simulink model "Parametrica"  (R2020b)
settings: Solver=VariableStepAuto  StartTime=0.0  StopTime=Smi.general.simulation_time  FixedStep=0.001  MaxStep=0.001  RelTol=1e-3  AbsTol=1e-3  EnableMultiTasking=on
undefined symbols (not defined in the file or in its folder): Smi, X, Y, Z
libraries: sm_lib x755, nesl_utility x196, simulink x8, dspsrcs4 x8, cstblocks x8
(part 6 of 26)

== system Parametrica/FIXED CHASSIS/WORLD ==
  Mechanism Configuration : sm_lib/Utilities/Mechanism Configuration  UniformGravity=Constant  GravityVector=[0 0 -9.80665]  GravityVectorUnits=m/s^2  GravityUnits=m/s^2  LinearizationDelta=0.001  JointModeTransitionNonlinearIterations=2
      settings: SourceProductName=Multibody
  Solver Configuration : nesl_utility/Solver Configuration  PhysicalDomain=network_engine_domain  SubClassName=solver  LeftPortType=input  RightPortType=generic  Tones=[]  Harmonics=[]  SimulateNoise=off  Profile=off  UseLocalSampling=off  EnableSwitchedLinearOptims=on  FrequencyDomain=off  UseCCode=off  RelTol=0.001  AbsTol=1e-06  MinStep=1e-09  ToWorkspace=off  RevertToSquareIcSolve=off  NumHomotopyIterations=100  PhasorMode=off  PhasorModeNumHarmonics=1  DoDC=off  ResidualTolerance=1e-09  UseLocalSolver=off  LocalSolverChoice=NE_BACKWARD_EULER_ADVANCER  LocalSolverSampleTime=0.001  DoFixedCost=off  MaxNonlinIter=3  MaxModeIter=2  ComputeImpulses=off  ImpulseIterations=2  LinearAlgebra=Sparse  EquationFormulation=NE_TIME_EF  DelaysMemoryBudget=1024  AutomaticFiltering=on  FilteringTimeConstant=0.001  PartitionStorageMethod=AS_NEEDED  PartitionMemoryBudget=1024  PartitionMethod=FAST
      settings: SourceProductName=Utilities
  World Frame : sm_lib/Frames and Transforms/World Frame
      settings: SourceProductName=Multibody
  WORLD : PMIOPort  Side=Right
  connections:
  WORLD/RConn1 -- Solver Configuration/RConn1 -- Mechanism Configuration/RConn1 -- World Frame/RConn1

== system Parametrica/MOVING CHASSIS/ACTUATOR FL ==
  ACTUATOR : Subsystem
  ACTUATOR IN/OUT : Subsystem
  OUTER ACTUATOR : Subsystem
      settings: PortSchema="{\"entries\":[{\"content\":{\"sides\":[{\"content\":{\"connectorIds\":[]},\"type\":\"ConnectorPlacement.EquallySpacedRectSide\",\"uuid\":\"d7e62bfe-6450-4a39-85d3-bed3049c321c\"},{\"content\":{\"connectorIds\":[],\"side\":\"RIGHT\"},\"type\":\"ConnectorPlacement.EquallySpacedRectSide\",\"uuid\":\"3cbc563a-0112-4986-bd57-0cf817b4d4bf\"},{\"content\":{\"connectorIds\":[\"LConn1\"],\"side\":\"TOP\"},\"type\":\"ConnectorPlacement.EquallySpacedRectSide\",\"uuid\":\"eb91a932-1d66-4430-a168-6ec694e02ce0\"},{\"content\":{\"connectorIds\":[\"RConn1\"],\"side\":\"BOTTOM\"},\"type\":\"ConnectorPlacement.EquallySpacedRectSide\",\"uuid\":\"a5a9eb1a-4070-480d-a72b-be2caa4d4ddd\"},{\"content\":{\"connectorIds\":[],\"side\":\"HIDDEN\"},\"type\":\"ConnectorPlacement.EquallySpacedRectSide\",\"uuid\":\"1c33bc41-55ff-4930-aaf8-325eabd2d214\"}]},\"type\":\"ConnectorPlacement.EquallySpacedConnector\",\"uuid\":\"9fea4cfe-800a-4673-925c-b7963aa13243\"}],\"packageUris\":[\"http://schema.mathworks.com/mf0/Connector/R2020b\"],\"version\":\"1.0\"}"
  Full geometry : PMIOPort  Side=Left
  WORLD : PMIOPort  Port=2  Side=Right
  CP : PMIOPort  Port=3  Side=Left
  connections:
  ACTUATOR/LConn1 -- Full geometry/RConn1
  ACTUATOR/LConn2 -- CP/RConn1
  OUTER ACTUATOR/LConn1 -- ACTUATOR IN/OUT/RConn1
  OUTER ACTUATOR/RConn1 -- WORLD/RConn1
  ACTUATOR IN/OUT/LConn1 -- ACTUATOR/RConn1

== system Parametrica/MOVING CHASSIS/ACTUATOR FR ==
  ACTUATOR : Subsystem
  ACTUATOR IN/OUT : Subsystem
  OUTER ACTUATOR : Subsystem
      settings: PortSchema="{\"entries\":[{\"content\":{\"sides\":[{\"content\":{\"connectorIds\":[]},\"type\":\"ConnectorPlacement.EquallySpacedRectSide\",\"uuid\":\"d7e62bfe-6450-4a39-85d3-bed3049c321c\"},{\"content\":{\"connectorIds\":[],\"side\":\"RIGHT\"},\"type\":\"ConnectorPlacement.EquallySpacedRectSide\",\"uuid\":\"3cbc563a-0112-4986-bd57-0cf817b4d4bf\"},{\"content\":{\"connectorIds\":[\"LConn1\"],\"side\":\"TOP\"},\"type\":\"ConnectorPlacement.EquallySpacedRectSide\",\"uuid\":\"eb91a932-1d66-4430-a168-6ec694e02ce0\"},{\"content\":{\"connectorIds\":[\"RConn1\"],\"side\":\"BOTTOM\"},\"type\":\"ConnectorPlacement.EquallySpacedRectSide\",\"uuid\":\"a5a9eb1a-4070-480d-a72b-be2caa4d4ddd\"},{\"content\":{\"connectorIds\":[],\"side\":\"HIDDEN\"},\"type\":\"ConnectorPlacement.EquallySpacedRectSide\",\"uuid\":\"1c33bc41-55ff-4930-aaf8-325eabd2d214\"}]},\"type\":\"ConnectorPlacement.EquallySpacedConnector\",\"uuid\":\"9fea4cfe-800a-4673-925c-b7963aa13243\"}],\"packageUris\":[\"http://schema.mathworks.com/mf0/Connector/R2020b\"],\"version\":\"1.0\"}"
  Full geometry : PMIOPort  Side=Left
  WORLD : PMIOPort  Port=2  Side=Right
  CP : PMIOPort  Port=3  Side=Left
  connections:
  ACTUATOR IN/OUT/LConn1 -- ACTUATOR/RConn1
  OUTER ACTUATOR/RConn1 -- WORLD/RConn1
  OUTER ACTUATOR/LConn1 -- ACTUATOR IN/OUT/RConn1
  ACTUATOR/LConn2 -- CP/RConn1
  ACTUATOR/LConn1 -- Full geometry/RConn1

== system Parametrica/MOVING CHASSIS/ACTUATOR RL ==
  ACTUATOR : Subsystem
  ACTUATOR IN/OUT : Subsystem
  OUTER ACTUATOR : Subsystem
      settings: PortSchema="{\"entries\":[{\"content\":{\"sides\":[{\"content\":{\"connectorIds\":[]},\"type\":\"ConnectorPlacement.EquallySpacedRectSide\",\"uuid\":\"d7e62bfe-6450-4a39-85d3-bed3049c321c\"},{\"content\":{\"connectorIds\":[],\"side\":\"RIGHT\"},\"type\":\"ConnectorPlacement.EquallySpacedRectSide\",\"uuid\":\"3cbc563a-0112-4986-bd57-0cf817b4d4bf\"},{\"content\":{\"connectorIds\":[\"LConn1\"],\"side\":\"TOP\"},\"type\":\"ConnectorPlacement.EquallySpacedRectSide\",\"uuid\":\"eb91a932-1d66-4430-a168-6ec694e02ce0\"},{\"content\":{\"connectorIds\":[\"RConn1\"],\"side\":\"BOTTOM\"},\"type\":\"ConnectorPlacement.EquallySpacedRectSide\",\"uuid\":\"a5a9eb1a-4070-480d-a72b-be2caa4d4ddd\"},{\"content\":{\"connectorIds\":[],\"side\":\"HIDDEN\"},\"type\":\"ConnectorPlacement.EquallySpacedRectSide\",\"uuid\":\"1c33bc41-55ff-4930-aaf8-325eabd2d214\"}]},\"type\":\"ConnectorPlacement.EquallySpacedConnector\",\"uuid\":\"9fea4cfe-800a-4673-925c-b7963aa13243\"}],\"packageUris\":[\"http://schema.mathworks.com/mf0/Connector/R2020b\"],\"version\":\"1.0\"}"
  Full geometry : PMIOPort  Side=Left
  WORLD : PMIOPort  Port=2  Side=Right
  CP : PMIOPort  Port=3  Side=Left
  connections:
  ACTUATOR IN/OUT/LConn1 -- ACTUATOR/RConn1
  OUTER ACTUATOR/RConn1 -- WORLD/RConn1
  OUTER ACTUATOR/LConn1 -- ACTUATOR IN/OUT/RConn1
  ACTUATOR/LConn2 -- CP/RConn1
  ACTUATOR/LConn1 -- Full geometry/RConn1

== system Parametrica/MOVING CHASSIS/ACTUATOR RR ==
  ACTUATOR : Subsystem
  ACTUATOR IN/OUT : Subsystem
  OUTER ACTUATOR : Subsystem
      settings: PortSchema="{\"entries\":[{\"content\":{\"sides\":[{\"content\":{\"connectorIds\":[]},\"type\":\"ConnectorPlacement.EquallySpacedRectSide\",\"uuid\":\"d7e62bfe-6450-4a39-85d3-bed3049c321c\"},{\"content\":{\"connectorIds\":[],\"side\":\"RIGHT\"},\"type\":\"ConnectorPlacement.EquallySpacedRectSide\",\"uuid\":\"3cbc563a-0112-4986-bd57-0cf817b4d4bf\"},{\"content\":{\"connectorIds\":[\"LConn1\"],\"side\":\"TOP\"},\"type\":\"ConnectorPlacement.EquallySpacedRectSide\",\"uuid\":\"eb91a932-1d66-4430-a168-6ec694e02ce0\"},{\"content\":{\"connectorIds\":[\"RConn1\"],\"side\":\"BOTTOM\"},\"type\":\"ConnectorPlacement.EquallySpacedRectSide\",\"uuid\":\"a5a9eb1a-4070-480d-a72b-be2caa4d4ddd\"},{\"content\":{\"connectorIds\":[],\"side\":\"HIDDEN\"},\"type\":\"ConnectorPlacement.EquallySpacedRectSide\",\"uuid\":\"1c33bc41-55ff-4930-aaf8-325eabd2d214\"}]},\"type\":\"ConnectorPlacement.EquallySpacedConnector\",\"uuid\":\"9fea4cfe-800a-4673-925c-b7963aa13243\"}],\"packageUris\":[\"http://schema.mathworks.com/mf0/Connector/R2020b\"],\"version\":\"1.0\"}"
  Full geometry : PMIOPort  Side=Left
  WORLD : PMIOPort  Port=2  Side=Right
  CP : PMIOPort  Port=3  Side=Left
  connections:
  ACTUATOR/LConn1 -- Full geometry/RConn1
  ACTUATOR/LConn2 -- CP/RConn1
  OUTER ACTUATOR/LConn1 -- ACTUATOR IN/OUT/RConn1
  OUTER ACTUATOR/RConn1 -- WORLD/RConn1
  ACTUATOR IN/OUT/LConn1 -- ACTUATOR/RConn1

== system Parametrica/MOVING CHASSIS/ARB FORCE FRONT1 ==
  ARB° LEFT : Inport
  ARB° RIGHT : Inport  Port=2
  Constant : Constant  Value=Smi.Car.FRONT.elastic.ARB_stiffness
  Product : Product
  Simulink-PS Converter : nesl_utility/Simulink-PS Converter  PhysicalDomain=network_engine_domain  SubClassName=ps_input  LeftPortType=input  RightPortType=output  PseudoPeriodic=off  Frequencies=[]  NoiseDistribution=none  NoiseParameters=[]  Unit=1  AffineConversion=off  FilteringAndDerivatives=provide  SimscapeFilterOrder=1  InputFilterTimeConstant=0.001  UdotUserProvided=0
  Sum : Sum  Inputs=+-
  ARB FORCE : PMIOPort  Side=Right
  wires:
  Sum/1 -> Product/1
  ARB° RIGHT/1 -> Sum/2
  ARB° LEFT/1 -> Sum/1
  Constant/1 -> Product/2
  Product/1 -> Simulink-PS Converter/1
  connections:
  ARB FORCE/RConn1 -- Simulink-PS Converter/RConn1

== system Parametrica/MOVING CHASSIS/ARB FORCE REAR ==
  ARB° LEFT : Inport
  ARB° RIGHT : Inport  Port=2
  Constant : Constant  Value=Smi.Car.REAR.elastic.ARB_stiffness
  Gain : Gain  Gain=180/pi
  Product : Product
  Scope : Scope
  Simulink-PS Converter : nesl_utility/Simulink-PS Converter  PhysicalDomain=network_engine_domain  SubClassName=ps_input  LeftPortType=input  RightPortType=output  PseudoPeriodic=off  Frequencies=[]  NoiseDistribution=none  NoiseParameters=[]  Unit=1  AffineConversion=off  FilteringAndDerivatives=provide  SimscapeFilterOrder=1  InputFilterTimeConstant=0.001  UdotUserProvided=0
  Sum : Sum  Inputs=+-
  ARB FORCE : PMIOPort  Side=Left
  wires:
  Product/1 -> Simulink-PS Converter/1
  Constant/1 -> Product/2
  ARB° LEFT/1 -> Sum/1
  ARB° RIGHT/1 -> Sum/2
  Sum/1 -> Gain/1, Product/1
  Gain/1 -> Scope/1
  connections:
  ARB FORCE/RConn1 -- Simulink-PS Converter/RConn1

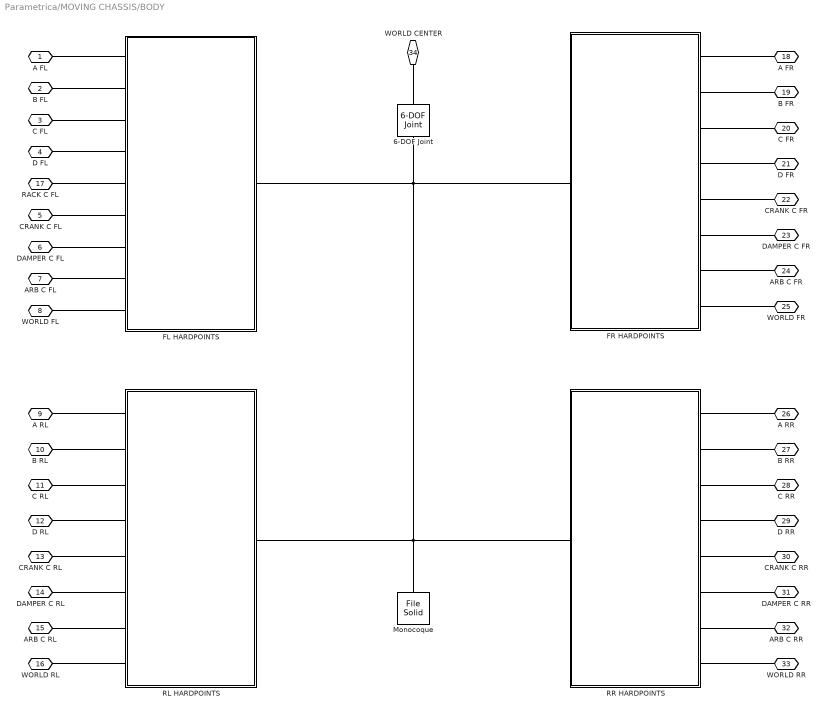
== system Parametrica/MOVING CHASSIS/BODY ==
  6-DOF Joint : sm_lib/Joints/6-DOF Joint  JointMode=Normal  SenseConstraintForce=off  SenseConstraintForceX=off  SenseConstraintForceY=off  SenseConstraintForceZ=off  SenseConstraintTorque=off  SenseConstraintTorqueX=off  SenseConstraintTorqueY=off  SenseConstraintTorqueZ=off  SenseTotalForce=off  SenseTotalForceX=off  SenseTotalForceY=off  SenseTotalForceZ=off  SenseTotalTorque=off  SenseTotalTorqueX=off  SenseTotalTorqueY=off  SenseTotalTorqueZ=off  CompositeWrenchDir=FollowerOnBase  CompositeWrenchFrame=BaseFrame  PxEquilibriumPosition=0  PxEquilibriumPositionUnits=m  PxSpringStiffness=0  PxSpringStiffnessUnits=N/m  PxDampingCoefficient=0  PxDampingCoefficientUnits=N/(m/s)  PxTorqueActuationMode=NoTorque  PxMotionActuationMode=ComputedMotion  PxSensePosition=off  PxSenseVelocity=off  PxSenseAcceleration=off  PxSenseTorqueForce=off  PxSenseLowerLimitTorqueForce=off  PxSenseUpperLimitTorqueForce=off  PxLowerLimitSpecify=off  PxLowerLimitBound=-1  PxLowerLimitBoundUnits=m  PxLowerLimitStiffness=1e6  PxLowerLimitStiffnessUnits=N/m  PxLowerLimitDamping=1e3  PxLowerLimitDampingUnits=N/(m/s)  PxLowerLimitTransitionRegionWidth=1e-4  PxLowerLimitTransitionRegionWidthUnits=m  PxUpperLimitSpecify=off  PxUpperLimitBound=1  PxUpperLimitBoundUnits=m  PxUpperLimitStiffness=1e6  PxUpperLimitStiffnessUnits=N/m  PxUpperLimitDamping=1e3  PxUpperLimitDampingUnits=N/(m/s)  PxUpperLimitTransitionRegionWidth=1e-4  PxUpperLimitTransitionRegionWidthUnits=m  PxPositionTargetSpecify=off  PxPositionTargetPriority=High  PxPositionTargetValue=0  PxPositionTargetValueUnits=m  PxVelocityTargetSpecify=off  PxVelocityTargetPriority=High  PxVelocityTargetValue=0  PxVelocityTargetValueUnits=m/s  PyEquilibriumPosition=0  PyEquilibriumPositionUnits=m  PySpringStiffness=0  PySpringStiffnessUnits=N/m  PyDampingCoefficient=0  PyDampingCoefficientUnits=N/(m/s)  PyTorqueActuationMode=NoTorque  PyMotionActuationMode=ComputedMotion  PySensePosition=off  PySenseVelocity=off  PySenseAcceleration=off  PySenseTorqueForce=off  PySenseLowerLimitTorqueForce=off  PySenseUpperLimitTorqueForce=off  PyLowerLimitSpecify=off  PyLowerLimitBound=-1  PyLowerLimitBoundUnits=m  PyLowerLimitStiffness=1e6  PyLowerLimitStiffnessUnits=N/m  PyLowerLimitDamping=1e3  PyLowerLimitDampingUnits=N/(m/s)  PyLowerLimitTransitionRegionWidth=1e-4  PyLowerLimitTransitionRegionWidthUnits=m  PyUpperLimitSpecify=off  PyUpperLimitBound=1  PyUpperLimitBoundUnits=m  PyUpperLimitStiffness=1e6  PyUpperLimitStiffnessUnits=N/m  PyUpperLimitDamping=1e3  PyUpperLimitDampingUnits=N/(m/s)  PyUpperLimitTransitionRegionWidth=1e-4  PyUpperLimitTransitionRegionWidthUnits=m  PyPositionTargetSpecify=off  PyPositionTargetPriority=High  PyPositionTargetValue=0  PyPositionTargetValueUnits=m  PyVelocityTargetSpecify=off  PyVelocityTargetPriority=High  PyVelocityTargetValue=0  PyVelocityTargetValueUnits=m/s  PzEquilibriumPosition=0  PzEquilibriumPositionUnits=m  PzSpringStiffness=0  PzSpringStiffnessUnits=N/m  PzDampingCoefficient=0  PzDampingCoefficientUnits=N/(m/s)  PzTorqueActuationMode=NoTorque  PzMotionActuationMode=ComputedMotion  PzSensePosition=off  PzSenseVelocity=off  PzSenseAcceleration=off  PzSenseTorqueForce=off  PzSenseLowerLimitTorqueForce=off  PzSenseUpperLimitTorqueForce=off  PzLowerLimitSpecify=off  PzLowerLimitBound=-1  PzLowerLimitBoundUnits=m  PzLowerLimitStiffness=1e6  PzLowerLimitStiffnessUnits=N/m  PzLowerLimitDamping=1e3  PzLowerLimitDampingUnits=N/(m/s)  PzLowerLimitTransitionRegionWidth=1e-4  PzLowerLimitTransitionRegionWidthUnits=m  PzUpperLimitSpecify=off  PzUpperLimitBound=1  PzUpperLimitBoundUnits=m  PzUpperLimitStiffness=1e6  PzUpperLimitStiffnessUnits=N/m  PzUpperLimitDamping=1e3  PzUpperLimitDampingUnits=N/(m/s)  PzUpperLimitTransitionRegionWidth=1e-4  PzUpperLimitTransitionRegionWidthUnits=m  PzPositionTargetSpecify=off  PzPositionTargetPriority=High  PzPositionTargetValue=0  PzPositionTargetValueUnits=m  PzVelocityTargetSpecify=off  PzVelocityTargetPriority=High  PzVelocityTargetValue=0  PzVelocityTargetValueUnits=m/s  SphDefPosRotationMethod=None  SphDefPosRotationAngleUnits=deg  SphDefPosRotationStandardAxis=+Z  SphDefPosRotationAngle=0.0  SphDefPosRotationArbitraryAxis=[0 0 1]  SphDefPosFollAlignAxisA=+X  SphDefPosBaseAlignAxisA=+Y  SphDefPosFollAlignAxisB=+Y  SphDefPosBaseAlignAxisB=+Z  SphDefPosRotationSequenceAxes=FollowerAxes  SphDefPosRotationSequence=XYX  SphDefPosRotationSequenceAngles=[0 0 0]  SphDefPosRotationSequenceAnglesUnits=deg  SphDefPosRotationMatrix=[1 0 0; 0 1 0; 0 0 1]  SphEqPosRotationMethod=None  SphEqPosRotationAngleUnits=deg  SphEqPosRotationStandardAxis=+Z  SphEqPosRotationAngle=0.0  SphEqPosRotationArbitraryAxis=[0 0 1]  SphEqPosFollAlignAxisA=+X  SphEqPosBaseAlignAxisA=+Y  SphEqPosFollAlignAxisB=+Y  SphEqPosBaseAlignAxisB=+Z  SphEqPosRotationSequenceAxes=FollowerAxes  SphEqPosRotationSequence=XYX  SphEqPosRotationSequenceAngles=[0 0 0]  SphEqPosRotationSequenceAnglesUnits=deg  SphEqPosRotationMatrix=[1 0 0; 0 1 0; 0 0 1]  SphSpringStiffness=0  SphSpringStiffnessUnits=N*m/deg  SphDampingCoefficient=0  SphDampingCoefficientUnits=N*m/(deg/s)  SphActuateTorqueX=off  SphActuateTorqueY=off  SphActuateTorqueZ=off  SphActuateTorque=off  SphTorqueActuationMode=NoTorque  SphMotionActuationMode=ComputedMotion  SphActuationFrame=BaseFrame  SphSensePosition=off  SphSenseVelocityX=off  SphSenseVelocityY=off  SphSenseVelocityZ=off  SphSenseVelocity=off  SphSenseAccelerationX=off  SphSenseAccelerationY=off  SphSenseAccelerationZ=off  SphSenseAcceleration=off  SphSenseTorqueX=off  SphSenseTorqueY=off  SphSenseTorqueZ=off  SphSenseTorqueForce=off  SphSenseLowerLimitTorqueMag=off  SphSenseUpperLimitTorqueMag=off  SphSensingFrame=BaseFrame  SphLowerLimitSpecify=off  SphLowerLimitBound=15  SphLowerLimitBoundUnits=deg  SphLowerLimitStiffness=1e4  SphLowerLimitStiffnessUnits=N*m/deg  SphLowerLimitDamping=10  SphLowerLimitDampingUnits=N*m/(deg/s)  SphLowerLimitTransitionRegionWidth=0.1  SphLowerLimitTransitionRegionWidthUnits=deg  SphUpperLimitSpecify=off  SphUpperLimitBound=45  SphUpperLimitBoundUnits=deg  SphUpperLimitStiffness=1e4  SphUpperLimitStiffnessUnits=N*m/deg  SphUpperLimitDamping=10  SphUpperLimitDampingUnits=N*m/(deg/s)  SphUpperLimitTransitionRegionWidth=0.1  SphUpperLimitTransitionRegionWidthUnits=deg  SphPositionTargetRotationMethod=None  SphPositionTargetRotationAngleUnits=deg  SphPositionTargetRotationStandardAxis=+Z  SphPositionTargetRotationAngle=0.0  SphPositionTargetRotationArbitraryAxis=[0 0 1]  SphPositionTargetFollAlignAxisA=+X  SphPositionTargetBaseAlignAxisA=+Y  SphPositionTargetFollAlignAxisB=+Y  SphPositionTargetBaseAlignAxisB=+Z  SphPositionTargetRotationSequenceAxes=FollowerAxes  SphPositionTargetRotationSequence=XYX  SphPositionTargetRotationSequenceAngles=[0 0 0]  SphPositionTargetRotationSequenceAnglesUnits=deg  SphPositionTargetRotationMatrix=[1 0 0; 0 1 0; 0 0 1]  SphPositionTargetSpecify=off  SphPositionTargetPriority=High  SphVelocityTargetValue=[0 0 0]  SphVelocityTargetValueUnits=deg/s  SphVelocityTargetSpecify=off  SphVelocityTargetPriority=High  SphVelocityTargetInFollowerFrame=on
  FL HARDPOINTS : Subsystem
  FR HARDPOINTS : Subsystem
  Monocoque : sm_lib/Body Elements/File Solid  ExtGeomFileName=Parameters\Monocoque.stp  UnitType=FromFile  ExtGeomFileUnits=m  StepReaderType=HEX  ExportConvexHullGeometry=off  InertiaType=PointMass  Mass=1  MassUnits=kg  CenterOfMass=[0 0 0]  CenterOfMassUnits=m  MomentsOfInertia=[1 1 1]  MomentsOfInertiaUnits=kg*m^2  ProductsOfInertia=[0 0 0]  ProductsOfInertiaUnits=kg*m^2  BasedOnType=DensityFromFile  Density=1000  DensityUnits=kg/m^3  DoExposeReferenceFrame=on  SerializedFrames=<Frames/>  GraphicType=FromGeometry  MarkerShape=Sphere  MarkerSize=10  GraphicVisPropType=SimpleVisualProperties  GraphicDiffuseColor=[1.0 1.0 1.0]  GraphicSpecularColor=[0.5 0.5 0.5 1.0]  GraphicAmbientColor=[0.15 0.15 0.15 1.0]  GraphicEmissiveColor=[0.0 0.0 0.0 1.0]  GraphicShininess=75  GraphicOpacity=0.4
  RL HARDPOINTS : Subsystem
  RR HARDPOINTS : Subsystem
  A FL : PMIOPort  Side=Left
  B FL : PMIOPort  Port=2  Side=Left
  C FL : PMIOPort  Port=3  Side=Left
  D FL : PMIOPort  Port=4  Side=Left
  CRANK C FL : PMIOPort  Port=5  Side=Left
  DAMPER C FL : PMIOPort  Port=6  Side=Left
  ARB C FL : PMIOPort  Port=7  Side=Left
  WORLD FL : PMIOPort  Port=8  Side=Left
  A RL : PMIOPort  Port=9  Side=Left
  B RL : PMIOPort  Port=10  Side=Left
  C RL : PMIOPort  Port=11  Side=Left
  D RL : PMIOPort  Port=12  Side=Left
  CRANK C RL : PMIOPort  Port=13  Side=Left
  DAMPER C RL : PMIOPort  Port=14  Side=Left
  ARB C RL : PMIOPort  Port=15  Side=Left
  WORLD RL : PMIOPort  Port=16  Side=Left
  RACK C FL : PMIOPort  Port=17  Side=Left
  A FR : PMIOPort  Port=18  Side=Right
  B FR : PMIOPort  Port=19  Side=Right
  C FR : PMIOPort  Port=20  Side=Right
  D FR : PMIOPort  Port=21  Side=Right
  CRANK C FR : PMIOPort  Port=22  Side=Right
  DAMPER C FR : PMIOPort  Port=23  Side=Right
  ARB C FR : PMIOPort  Port=24  Side=Right
  WORLD FR : PMIOPort  Port=25  Side=Right
  A RR : PMIOPort  Port=26  Side=Right
  B RR : PMIOPort  Port=27  Side=Right
  C RR : PMIOPort  Port=28  Side=Right
  D RR : PMIOPort  Port=29  Side=Right
  CRANK C RR : PMIOPort  Port=30  Side=Right
  DAMPER C RR : PMIOPort  Port=31  Side=Right
  ARB C RR : PMIOPort  Port=32  Side=Right
  WORLD RR : PMIOPort  Port=33  Side=Right
  WORLD CENTER : PMIOPort  Port=34  Side=Right
  connections:
  FL HARDPOINTS/RConn1 -- 6-DOF Joint/RConn1 -- RL HARDPOINTS/RConn1 -- Monocoque/RConn1 -- RR HARDPOINTS/RConn1 -- FR HARDPOINTS/RConn1
  A FL/RConn1 -- FL HARDPOINTS/LConn1
  B FL/RConn1 -- FL HARDPOINTS/LConn2
  C FL/RConn1 -- FL HARDPOINTS/LConn3
  D FL/RConn1 -- FL HARDPOINTS/LConn4
  RACK C FL/RConn1 -- FL HARDPOINTS/LConn5
  CRANK C FL/RConn1 -- FL HARDPOINTS/LConn6
  FL HARDPOINTS/LConn7 -- DAMPER C FL/RConn1
  FL HARDPOINTS/LConn8 -- ARB C FL/RConn1
  FL HARDPOINTS/LConn9 -- WORLD FL/RConn1
  FR HARDPOINTS/LConn8 -- WORLD FR/RConn1
  FR HARDPOINTS/LConn7 -- ARB C FR/RConn1
  FR HARDPOINTS/LConn6 -- DAMPER C FR/RConn1
  D FR/RConn1 -- FR HARDPOINTS/LConn4
  B FR/RConn1 -- FR HARDPOINTS/LConn2
  C FR/RConn1 -- FR HARDPOINTS/LConn3
  CRANK C FR/RConn1 -- FR HARDPOINTS/LConn5
  A FR/RConn1 -- FR HARDPOINTS/LConn1
  RL HARDPOINTS/LConn8 -- WORLD RL/RConn1
  RL HARDPOINTS/LConn7 -- ARB C RL/RConn1
  CRANK C RL/RConn1 -- RL HARDPOINTS/LConn5
  RL HARDPOINTS/LConn6 -- DAMPER C RL/RConn1
  D RL/RConn1 -- RL HARDPOINTS/LConn4
  C RL/RConn1 -- RL HARDPOINTS/LConn3
  B RL/RConn1 -- RL HARDPOINTS/LConn2
  A RL/RConn1 -- RL HARDPOINTS/LConn1
  A RR/RConn1 -- RR HARDPOINTS/LConn1
  C RR/RConn1 -- RR HARDPOINTS/LConn3
  CRANK C RR/RConn1 -- RR HARDPOINTS/LConn5
  D RR/RConn1 -- RR HARDPOINTS/LConn4
  B RR/RConn1 -- RR HARDPOINTS/LConn2
  RR HARDPOINTS/LConn7 -- ARB C RR/RConn1
  RR HARDPOINTS/LConn8 -- WORLD RR/RConn1
  RR HARDPOINTS/LConn6 -- DAMPER C RR/RConn1
  WORLD CENTER/RConn1 -- 6-DOF Joint/LConn1

== system Parametrica/MOVING CHASSIS/FIXED ACTUATORS ==
  FL HARDPOINTS : Subsystem
  FR HARDPOINTS : Subsystem
  RL HARDPOINTS : Subsystem
  RR HARDPOINTS : Subsystem
  OUTER ACTUATOR RL : PMIOPort  Side=Left
  OUTER ACTUATOR FL : PMIOPort  Port=2  Side=Left
  OUTER ACTUATOR RR : PMIOPort  Port=3  Side=Right
  OUTER ACTUATOR FR : PMIOPort  Port=4  Side=Right
  WORLD CENTER : PMIOPort  Port=5  Side=Right
  connections:
  FL HARDPOINTS/RConn1 -- RL HARDPOINTS/RConn1 -- RR HARDPOINTS/RConn1 -- WORLD CENTER/RConn1 -- FR HARDPOINTS/RConn1
  OUTER ACTUATOR FL/RConn1 -- FL HARDPOINTS/LConn1
  OUTER ACTUATOR FR/RConn1 -- FR HARDPOINTS/LConn1
  OUTER ACTUATOR RL/RConn1 -- RL HARDPOINTS/LConn1
  OUTER ACTUATOR RR/RConn1 -- RR HARDPOINTS/LConn1
